simulink model "gm_uz_JL_invModel_ideal"  (R2025a)
settings: Solver=FixedStepDiscrete  StartTime=0.0  StopTime=0.1  RelTol=1e-3
settings Model: SimulationMode=accelerator  Creator=jonat  LastModifiedBy=jonat
settings SolverCC: AlgebraicLoopSolver=TrustRegion
settings DataIOCC: LimitDataPoints=on  SaveOutput=off  SaveTime=off
settings OptimizationCC: BlockReduction=off  ConditionallyExecuteInputs=off  DefaultParameterBehavior=Inlined  LifeSpan=inf
settings DebuggingCC: AlgebraicLoopMsg=error  InheritedTsInSrcMsg=none  SingleTaskRateTransMsg=error  UnconnectedInputMsg=warning  UnconnectedOutputMsg=warning  UnconnectedLineMsg=warning  AllowSymbolicDim=off  StrictBusMsg=ErrorOnBusTreatedAsVector  SFUnexpectedBacktrackingDiag=warning  SFNoUnconditionalDefaultTransitionDiag=warning  SFExecutionAtInitializationDiag=none  ArithmeticOperatorsInVariantConditions=warning
settings HardwareCC: ProdBitPerPointer=32.0  ProdBitPerSizeT=32.0  ProdBitPerPtrDiffT=32.0  ProdLargestAtomicFloat=None  ProdIntDivRoundTo=Undefined  ProdEndianess=Unspecified  ProdWordSize=32.0  ProdHWDeviceType=ASIC/FPGA->ASIC/FPGA  ProdEqTarget=off
settings ModelReferenceCC: EnableRefExpFcnMdlSchedulingChecks=on
settings SFSimCC: SimUseLocalCustomCode=off  CustomCodeUndefinedFunction=UseInterfaceOnly
settings RTWCC: RTWUseLocalCustomCode=off  GPUComputeCapability=3.5
settings CodeAppCC: StateflowObjectComments=on
settings GRTTargetCC: TargetLangStandard=C89/C90 (ANSI)
settings ConfigComp: CovScope=ReferencedModels  CovMetricSettings=dw  CovSaveCumulativeToWorkspaceVar=on  CovSaveSingleToWorkspaceVar=on  CovExternalEMLEnable=off  CovSFcnEnable=off

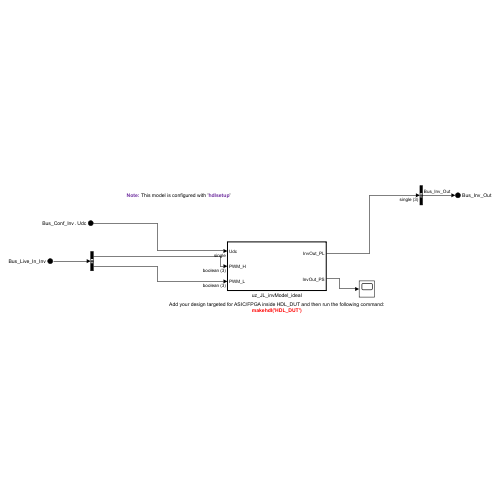
[thumbnail: Simulink's stored preview of the top-level diagram]
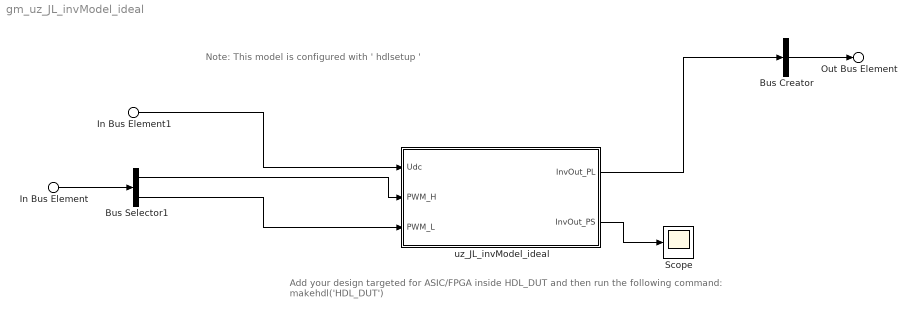
== system gm_uz_JL_invModel_ideal ==
  note: Add your design targeted for ASIC/FPGA inside HDL_DUT and then run the following command:
      | makehdl('HDL_DUT')
  note: Note: This model is configured with ' hdlsetup '
  In Bus Element : Inport  PortName=Bus_Live_In_Inv
  In Bus Element1 : Inport  Port=2  PortName=Bus_Conf_Inv  Element=Udc
  Bus Creator : BusCreator  Inputs=1  OutDataTypeStr=Bus: Bus_Inv_Out  NonVirtualBus=on
      settings: InheritFromInputs=off
  Bus Selector1 : BusSelector  OutputSignals=PWM_H,PWM_L
  Scope : Scope
      settings: ActiveDisplayYMinimum=-497.00837732959218  ActiveDisplayYMaximum=484.07881017040796
  uz_JL_invModel_ideal : Subsystem  TreatAsAtomicUnit=on
  Out Bus Element : Outport  PortName=Bus_Inv_Out
  wires:
  uz_JL_invModel_ideal/1(InvOut_PL) -> Bus Creator/1
  Bus Selector1/2 -> uz_JL_invModel_ideal/3(PWM_L)
  Bus Selector1/1 -> uz_JL_invModel_ideal/2(PWM_H)
  In Bus Element1/1 -> uz_JL_invModel_ideal/1(Udc)
  uz_JL_invModel_ideal/2(InvOut_PS) -> Scope/1
  Bus Creator/1 -> Out Bus Element/1
  In Bus Element/1 -> Bus Selector1/1

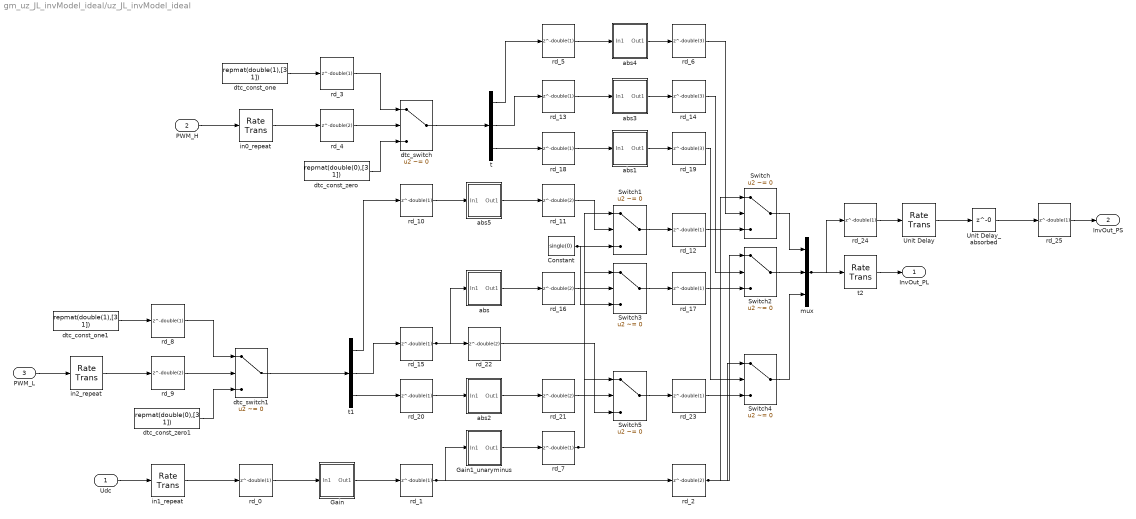
== system gm_uz_JL_invModel_ideal/uz_JL_invModel_ideal ==
  Udc : Inport  OutDataTypeStr=single  PortDimensions=1  SampleTime=0.002
  PWM_H : Inport  Port=2  OutDataTypeStr=boolean  PortDimensions=[3]  SampleTime=0.002
  PWM_L : Inport  Port=3  OutDataTypeStr=boolean  PortDimensions=[3]  SampleTime=0.002
  Constant : Constant  Value=single(0)  OutDataTypeStr=single  SampleTime=8e-05
  Gain : Subsystem
      mask Display: disp('NFP\ngain_pow2');
  Gain1_unaryminus : Subsystem
      mask Display: disp('NFP\numinus');
  Switch{,1..5} (6 alike) : Switch  Criteria=u2 ~= 0  Threshold=single(0)  OutDataTypeStr=single  SampleTime=8e-05  SaturateOnIntegerOverflow=off  InputSameDT=off
  Unit Delay : RateTransition  InitialCondition=double(0)  OutPortSampleTimeOpt=Multiple of input port sample time  OutPortSampleTimeMultiple=25
  Unit Delay_absorbed : Delay  DelayLength=0
  abs : Subsystem
      mask Display: disp('NFP\nabs');
  abs1 : Subsystem
      mask Display: disp('NFP\nabs');
  abs2 : Subsystem
      mask Display: disp('NFP\nabs');
  abs3 : Subsystem
      mask Display: disp('NFP\nabs');
  abs4 : Subsystem
      mask Display: disp('NFP\nabs');
  abs5 : Subsystem
      mask Display: disp('NFP\nabs');
  dtc_const_one : Constant  Value="repmat(double(1),[3  1])"  OutDataTypeStr=single  SampleTime=8e-05
  dtc_const_one1 : Constant  Value="repmat(double(1),[3  1])"  OutDataTypeStr=single  SampleTime=8e-05
  dtc_const_zero : Constant  Value="repmat(double(0),[3  1])"  OutDataTypeStr=single  SampleTime=8e-05
  dtc_const_zero1 : Constant  Value="repmat(double(0),[3  1])"  OutDataTypeStr=single  SampleTime=8e-05
  dtc_switch : Switch  Criteria=u2 ~= 0  Threshold=double(0)  OutDataTypeStr=single  SampleTime=8e-05  SaturateOnIntegerOverflow=off  InputSameDT=off
  dtc_switch1 : Switch  Criteria=u2 ~= 0  Threshold=double(0)  OutDataTypeStr=single  SampleTime=8e-05  SaturateOnIntegerOverflow=off  InputSameDT=off
  in0_repeat : RateTransition  Integrity=off  Deterministic=off  OutPortSampleTimeOpt=Multiple of input port sample time  OutPortSampleTimeMultiple=1/25
  in1_repeat : RateTransition  Integrity=off  Deterministic=off  OutPortSampleTimeOpt=Multiple of input port sample time  OutPortSampleTimeMultiple=1/25
  in2_repeat : RateTransition  Integrity=off  Deterministic=off  OutPortSampleTimeOpt=Multiple of input port sample time  OutPortSampleTimeMultiple=1/25
  mux : Mux  Inputs=3
  rd_{0..1,3,5,7..8,10,12..13,15,17..18,20,23..24} (15 alike) : Delay  DelayLength=double(1)  InitialCondition=0  SampleTime=8e-05
  rd_{2,4,9,11,16,21..22} (7 alike) : Delay  DelayLength=double(2)  InitialCondition=0  SampleTime=8e-05
  rd_14 : Delay  DelayLength=double(3)  InitialCondition=0  SampleTime=8e-05
  rd_19 : Delay  DelayLength=double(3)  InitialCondition=0  SampleTime=8e-05
  rd_25 : Delay  DelayLength=double(1)  InitialCondition=0  SampleTime=0.002
  rd_6 : Delay  DelayLength=double(3)  InitialCondition=0  SampleTime=8e-05
  t : Demux  Outputs=3
  t1 : Demux  Outputs=3
  t2 : RateTransition  InitialCondition=double(0)  OutPortSampleTimeOpt=Multiple of input port sample time  OutPortSampleTimeMultiple=25
  InvOut_PL : Outport  SampleTime=0.002
  InvOut_PS : Outport  Port=2  SampleTime=0.002
  wires:
  abs/1(Out1) -> rd_16/1
  Udc/1 -> in1_repeat/1
  dtc_const_zero1/1 -> dtc_switch1/3
  Switch1/1 -> rd_12/1
  PWM_L/1 -> in2_repeat/1
  dtc_const_one1/1 -> rd_8/1
  in2_repeat/1 -> rd_9/1
  rd_9/1 -> dtc_switch1/2
  in1_repeat/1 -> rd_0/1
  PWM_H/1 -> in0_repeat/1
  rd_8/1 -> dtc_switch1/1
  dtc_const_one/1 -> rd_3/1
  in0_repeat/1 -> rd_4/1
  mux/1 -> rd_24/1, t2/1
  dtc_switch1/1 -> t1/1
  rd_0/1 -> Gain/1(In1)
  rd_3/1 -> dtc_switch/1
  abs5/1(Out1) -> rd_11/1
  rd_4/1 -> dtc_switch/2
  dtc_const_zero/1 -> dtc_switch/3
  t1/1 -> rd_10/1
  t/3 -> rd_18/1
  t1/2 -> rd_15/1
  t1/3 -> rd_20/1
  Gain/1(Out1) -> rd_1/1
  Constant/1 -> Switch1/3, Switch3/3
  dtc_switch/1 -> t/1
  rd_10/1 -> abs5/1(In1)
  rd_15/1 -> rd_22/1, abs/1(In1)
  rd_20/1 -> abs2/1(In1)
  rd_1/1 -> rd_2/1, Gain1_unaryminus/1(In1)
  t/1 -> rd_5/1
  t/2 -> rd_13/1
  rd_22/1 -> Switch5/3
  abs2/1(Out1) -> rd_21/1
  Gain1_unaryminus/1(Out1) -> rd_7/1
  rd_5/1 -> abs4/1(In1)
  rd_13/1 -> abs3/1(In1)
  rd_18/1 -> abs1/1(In1)
  rd_11/1 -> Switch1/2
  rd_16/1 -> Switch3/2
  rd_21/1 -> Switch5/2
  rd_7/1 -> Switch5/1, Switch3/1, Switch1/1
  t2/1 -> InvOut_PL/1
  abs4/1(Out1) -> rd_6/1
  abs3/1(Out1) -> rd_14/1
  abs1/1(Out1) -> rd_19/1
  Switch3/1 -> rd_17/1
  Switch5/1 -> rd_23/1
  rd_6/1 -> Switch/2
  rd_14/1 -> Switch2/2
  rd_19/1 -> Switch4/2
  rd_12/1 -> Switch/3
  rd_17/1 -> Switch2/3
  rd_23/1 -> Switch4/3
  rd_2/1 -> Switch/1, Switch4/1, Switch2/1
  Switch/1 -> mux/1
  Switch2/1 -> mux/2
  Switch4/1 -> mux/3
  rd_24/1 -> Unit Delay/1
  Unit Delay/1 -> Unit Delay_absorbed/1
  Unit Delay_absorbed/1 -> rd_25/1
  rd_25/1 -> InvOut_PS/1

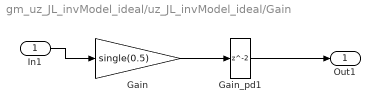
== system gm_uz_JL_invModel_ideal/uz_JL_invModel_ideal/Gain ==
  In1 : Inport
  Gain : Gain  Gain=single(0.5)
  Gain_pd1 : Delay
  Out1 : Outport
  wires:
  In1/1 -> Gain/1
  Gain/1 -> Gain_pd1/1
  Gain_pd1/1 -> Out1/1

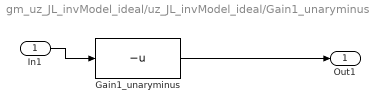
== system gm_uz_JL_invModel_ideal/uz_JL_invModel_ideal/Gain1_unaryminus ==
  In1 : Inport
  Gain1_unaryminus : UnaryMinus  SampleTime=8e-05
  Out1 : Outport
  wires:
  In1/1 -> Gain1_unaryminus/1
  Gain1_unaryminus/1 -> Out1/1

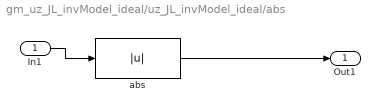
== system gm_uz_JL_invModel_ideal/uz_JL_invModel_ideal/abs ==
  In1 : Inport
  abs : Abs  SampleTime=8e-05  OutDataTypeStr=single  SaturateOnIntegerOverflow=off
  Out1 : Outport
  wires:
  In1/1 -> abs/1
  abs/1 -> Out1/1

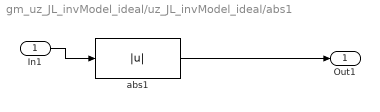
== system gm_uz_JL_invModel_ideal/uz_JL_invModel_ideal/abs1 ==
  In1 : Inport
  abs1 : Abs  SampleTime=8e-05  OutDataTypeStr=single  SaturateOnIntegerOverflow=off
  Out1 : Outport
  wires:
  In1/1 -> abs1/1
  abs1/1 -> Out1/1

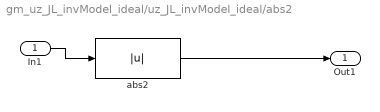
== system gm_uz_JL_invModel_ideal/uz_JL_invModel_ideal/abs2 ==
  In1 : Inport
  abs2 : Abs  SampleTime=8e-05  OutDataTypeStr=single  SaturateOnIntegerOverflow=off
  Out1 : Outport
  wires:
  In1/1 -> abs2/1
  abs2/1 -> Out1/1

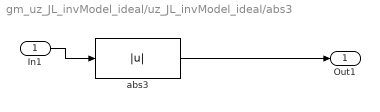
== system gm_uz_JL_invModel_ideal/uz_JL_invModel_ideal/abs3 ==
  In1 : Inport
  abs3 : Abs  SampleTime=8e-05  OutDataTypeStr=single  SaturateOnIntegerOverflow=off
  Out1 : Outport
  wires:
  In1/1 -> abs3/1
  abs3/1 -> Out1/1

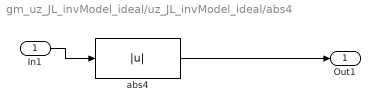
== system gm_uz_JL_invModel_ideal/uz_JL_invModel_ideal/abs4 ==
  In1 : Inport
  abs4 : Abs  SampleTime=8e-05  OutDataTypeStr=single  SaturateOnIntegerOverflow=off
  Out1 : Outport
  wires:
  In1/1 -> abs4/1
  abs4/1 -> Out1/1

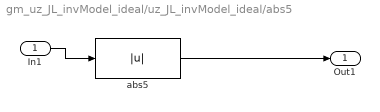
== system gm_uz_JL_invModel_ideal/uz_JL_invModel_ideal/abs5 ==
  In1 : Inport
  abs5 : Abs  SampleTime=8e-05  OutDataTypeStr=single  SaturateOnIntegerOverflow=off
  Out1 : Outport
  wires:
  In1/1 -> abs5/1
  abs5/1 -> Out1/1
